simulink model "inverter_hil"  (R2024b)
settings: Solver=FixedStepDiscrete  StartTime=0.0  StopTime=inf  FixedStep=0.001  RelTol=1e-3
InitFcn:
  | enforceHardwarePreflight(bdroot);
values from neighbouring files (symbols this model uses):
  hil_cal_pedals_pressed_v1 = 1.1631952391851683    [inverter_hil.sldd]
  hil_cal_pedals_pressed_v2 = 2.341496910048066    [inverter_hil.sldd]
  hil_cal_pedals_pressed_v3 = 1.6012817578393226    [inverter_hil.sldd]
  hil_cal_pedals_pressed_v4 = 1.6012817578393226    [inverter_hil.sldd]
  hil_cal_pedals_released_v1 = 1.5156786449988555    [inverter_hil.sldd]
  hil_cal_pedals_released_v2 = 3.2025635156786452    [inverter_hil.sldd]
  hil_cal_pedals_released_v3 = 0.45445181963836118    [inverter_hil.sldd]
  hil_cal_pedals_released_v4 = 0.45445181963836118    [inverter_hil.sldd]
  hil_cmd_can_drop_control_mask = 0    [inverter_hil.sldd]
  hil_cmd_can_drop_status_mask = 0    [inverter_hil.sldd]
  hil_cmd_dc_link12_v = 0.0    [inverter_hil.sldd]
  hil_cmd_dc_link34_v = 0.0    [inverter_hil.sldd]
  hil_cmd_digital_cooling_switch = 0    [inverter_hil.sldd]
  hil_cmd_digital_main_button = 0    [inverter_hil.sldd]
  hil_cmd_digital_main_button_sequence = 0    [inverter_hil.sldd]
  hil_cmd_digital_precharge_sequence = 0    [inverter_hil.sldd]
  hil_cmd_digital_shutdown_feedback = 0    [inverter_hil.sldd]
  hil_cmd_gui_heartbeat = 0    [inverter_hil.sldd]
  hil_cmd_imu_dropout = 0    [inverter_hil.sldd]
  hil_cmd_imu_malformed = 0    [inverter_hil.sldd]
  hil_cmd_imu_stale = 0    [inverter_hil.sldd]
  hil_cmd_inverter1_connected = 1    [inverter_hil.sldd]
  hil_cmd_inverter1_fault_mask = 0    [inverter_hil.sldd]
  hil_cmd_inverter1_load_nm = 0.0    [inverter_hil.sldd]
  hil_cmd_inverter2_connected = 1    [inverter_hil.sldd]
  hil_cmd_inverter2_fault_mask = 0    [inverter_hil.sldd]
  hil_cmd_inverter2_load_nm = 0.0    [inverter_hil.sldd]
  hil_cmd_inverter3_connected = 1    [inverter_hil.sldd]
  hil_cmd_inverter3_fault_mask = 0    [inverter_hil.sldd]
  hil_cmd_inverter3_load_nm = 0.0    [inverter_hil.sldd]
  hil_cmd_inverter4_connected = 1    [inverter_hil.sldd]
  hil_cmd_inverter4_fault_mask = 0    [inverter_hil.sldd]
  hil_cmd_inverter4_load_nm = 0.0    [inverter_hil.sldd]
  hil_cmd_pedals_brake = 0.0    [inverter_hil.sldd]
  hil_cmd_pedals_plausibility_override = 0    [inverter_hil.sldd]
  hil_cmd_pedals_throttle = 0.0    [inverter_hil.sldd]
  hil_cmd_steering_angle_deg = 0.0    [inverter_hil.sldd]
  hil_cmd_steering_angle_sentinel = 0    [inverter_hil.sldd]
  hil_cmd_steering_calibration_sequence = 0    [inverter_hil.sldd]
  hil_cmd_steering_dropout = 0    [inverter_hil.sldd]
  hil_cmd_steering_invalid_status = 0    [inverter_hil.sldd]
  hil_cmd_steering_malformed = 0    [inverter_hil.sldd]
  hil_cmd_steering_speed_sentinel = 0    [inverter_hil.sldd]
  hil_cmd_steering_stale = 0    [inverter_hil.sldd]
undefined symbols (not defined in the file or in its folder): Pull, up
libraries: speedgoatlib_IO614 x21, canmsglib x16, speedgoatlib_IO183 x5
(part 1 of 3)
settings Model: DataDictionary=inverter_hil.sldd  Creator=MFE-HPC  LastModifiedBy=MFE-HPC
settings SolverCC: ConcurrentTasks=on  PositivePriorityOrder=on
settings OptimizationCC: BlockReduction=off  OptimizeBlockIOStorage=off
settings DebuggingCC: TasksWithSamePriorityMsg=none
settings HardwareCC: ProdBitPerLong=64  ProdLongLongMode=on  ProdHWDeviceType=Intel->x86-64 (Linux 64)
settings RTWCC: Description=Speedgoat Real-Time Target Machine  SystemTargetFile=speedgoat.tlc  TemplateMakefile=slrealtime_default_tmf  Toolchain=Simulink Real-Time Toolchain  BuildConfiguration=Faster Runs  CodeExecutionProfiling=on  TargetLang=C++
settings SimulinkRealTimeTargetCC: InstructionSetFMA=off  LogToMDFFile=off

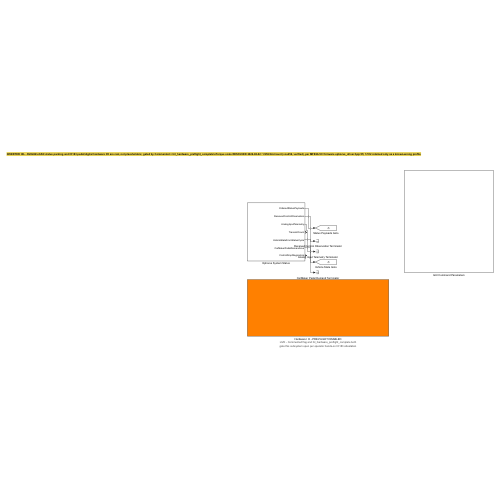
[thumbnail: Simulink's stored preview of the top-level diagram]
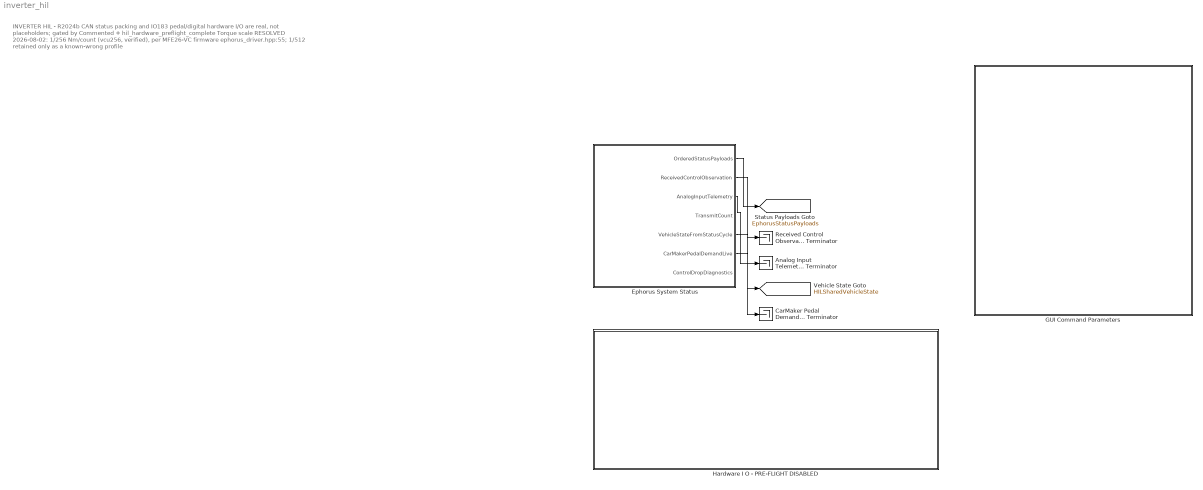
== system inverter_hil ==
  note: INVERTER HIL - R2024b\nCAN status packing and IO183 pedal/digital hardware I/O are real, not placeholders; gated by Commented + hil_hardware_preflight_complete\nTorque scale RESOLVED 2026-08-02: 1/256 Nm/count (vcu256, verified), per MFE26-VC firmware ephorus_driver.hpp:55; 1/512 retained only as a known-wrong profile
  Analog Input Telemetry Terminator : Terminator
  CarMaker Pedal Demand Terminator : Terminator
  Ephorus System Status : Subsystem
  GUI Command Parameters : Subsystem
  Hardware I O - PRE-FLIGHT DISABLED : Subsystem
      settings: AttributesFormatString=LIVE - Commented flag and hil_hardware_preflight_complete both\ngate this subsystem open per operator hands-on IO183 attestation
  Received Control Observation Terminator : Terminator
  tag scope: EphorusStatusPayloads=global, HILSharedVehicleState=global
  wires:
  Ephorus System Status/1(OrderedStatusPayloads) -> [EphorusStatusPayloads]
  Ephorus System Status/2(ReceivedControlObservation) -> Received Control Observation Terminator/1
  Ephorus System Status/3(AnalogInputTelemetry) -> Analog Input Telemetry Terminator/1
  Ephorus System Status/5(VehicleStateFromStatusCycle) -> [HILSharedVehicleState]
  Ephorus System Status/6(CarMakerPedalDemandLive) -> CarMaker Pedal Demand Terminator/1

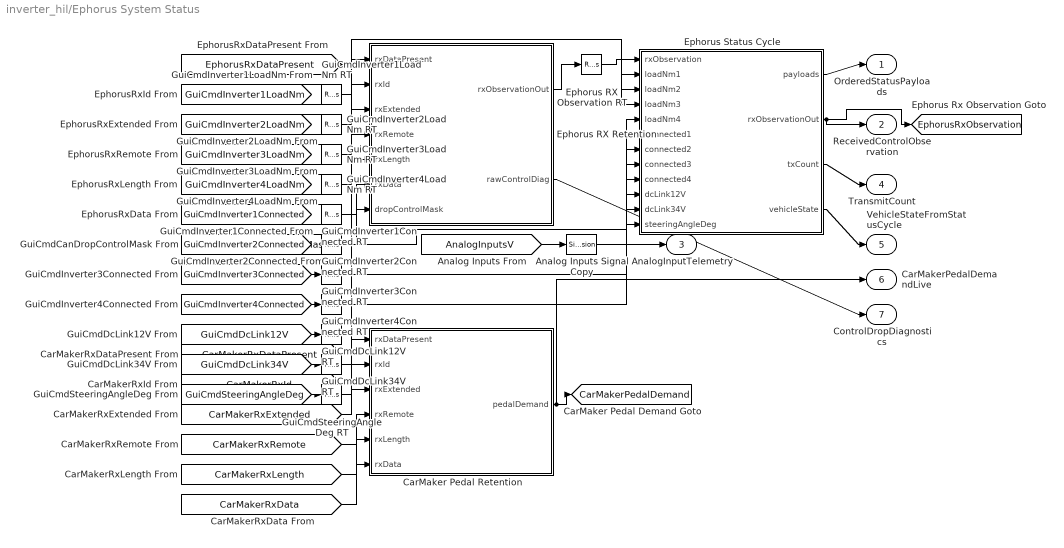
== system inverter_hil/Ephorus System Status ==
  Analog Inputs Signal Copy : SignalConversion  OverrideOpt=off
  CarMaker Pedal Retention : MATLAB Function  TreatAsAtomicUnit=on
  Ephorus RX Observation RT : RateTransition
  Ephorus RX Retention : MATLAB Function  TreatAsAtomicUnit=on
  Ephorus Status Cycle : MATLAB Function  TreatAsAtomicUnit=on
  GuiCmdDcLink12V RT : RateTransition
  GuiCmdDcLink34V RT : RateTransition
  GuiCmdInverter1Connected RT : RateTransition
  GuiCmdInverter1LoadNm RT : RateTransition
  GuiCmdInverter2Connected RT : RateTransition
  GuiCmdInverter2LoadNm RT : RateTransition
  GuiCmdInverter3Connected RT : RateTransition
  GuiCmdInverter3LoadNm RT : RateTransition
  GuiCmdInverter4Connected RT : RateTransition
  GuiCmdInverter4LoadNm RT : RateTransition
  GuiCmdSteeringAngleDeg RT : RateTransition
  OrderedStatusPayloads : Outport
  ReceivedControlObservation : Outport  Port=2
  AnalogInputTelemetry : Outport  Port=3
  TransmitCount : Outport  Port=4
  VehicleStateFromStatusCycle : Outport  Port=5
  CarMakerPedalDemandLive : Outport  Port=6
  ControlDropDiagnostics : Outport  Port=7
  tag scope: CarMakerPedalDemand=global, EphorusRxObservation=global
  wires:
  ? -> ?
  [EphorusRxDataPresent] -> Ephorus RX Retention/1(rxDataPresent)
  [EphorusRxId] -> Ephorus RX Retention/2(rxId)
  [EphorusRxExtended] -> Ephorus RX Retention/3(rxExtended)
  [EphorusRxRemote] -> Ephorus RX Retention/4(rxRemote)
  [EphorusRxLength] -> Ephorus RX Retention/5(rxLength)
  [EphorusRxData] -> Ephorus RX Retention/6(rxData)
  [GuiCmdCanDropControlMask] -> Ephorus RX Retention/7(dropControlMask)
  [CarMakerRxDataPresent] -> CarMaker Pedal Retention/1(rxDataPresent)
  [CarMakerRxId] -> CarMaker Pedal Retention/2(rxId)
  [CarMakerRxExtended] -> CarMaker Pedal Retention/3(rxExtended)
  [CarMakerRxRemote] -> CarMaker Pedal Retention/4(rxRemote)
  [CarMakerRxLength] -> CarMaker Pedal Retention/5(rxLength)
  [CarMakerRxData] -> CarMaker Pedal Retention/6(rxData)
  CarMaker Pedal Retention/1(pedalDemand) -> [CarMakerPedalDemand], CarMakerPedalDemandLive/1
  Ephorus RX Retention/1(rxObservationOut) -> Ephorus RX Observation RT/1
  Ephorus RX Observation RT/1 -> Ephorus Status Cycle/1(rxObservation)
  Ephorus Status Cycle/1(payloads) -> OrderedStatusPayloads/1
  Ephorus Status Cycle/2(rxObservationOut) -> ReceivedControlObservation/1, [EphorusRxObservation]
  Ephorus RX Retention/2(rawControlDiag) -> ControlDropDiagnostics/1
  [AnalogInputsV] -> Analog Inputs Signal Copy/1
  Analog Inputs Signal Copy/1 -> AnalogInputTelemetry/1
  Ephorus Status Cycle/3(txCount) -> TransmitCount/1
  Ephorus Status Cycle/4(vehicleState) -> VehicleStateFromStatusCycle/1
  [GuiCmdInverter1LoadNm] -> GuiCmdInverter1LoadNm RT/1
  GuiCmdInverter1LoadNm RT/1 -> Ephorus Status Cycle/2(loadNm1)
  [GuiCmdInverter2LoadNm] -> GuiCmdInverter2LoadNm RT/1
  GuiCmdInverter2LoadNm RT/1 -> Ephorus Status Cycle/3(loadNm2)
  [GuiCmdInverter3LoadNm] -> GuiCmdInverter3LoadNm RT/1
  GuiCmdInverter3LoadNm RT/1 -> Ephorus Status Cycle/4(loadNm3)
  [GuiCmdInverter4LoadNm] -> GuiCmdInverter4LoadNm RT/1
  GuiCmdInverter4LoadNm RT/1 -> Ephorus Status Cycle/5(loadNm4)
  [GuiCmdInverter1Connected] -> GuiCmdInverter1Connected RT/1
  GuiCmdInverter1Connected RT/1 -> Ephorus Status Cycle/6(connected1)
  [GuiCmdInverter2Connected] -> GuiCmdInverter2Connected RT/1
  GuiCmdInverter2Connected RT/1 -> Ephorus Status Cycle/7(connected2)
  [GuiCmdInverter3Connected] -> GuiCmdInverter3Connected RT/1
  GuiCmdInverter3Connected RT/1 -> Ephorus Status Cycle/8(connected3)
  [GuiCmdInverter4Connected] -> GuiCmdInverter4Connected RT/1
  GuiCmdInverter4Connected RT/1 -> Ephorus Status Cycle/9(connected4)
  [GuiCmdDcLink12V] -> GuiCmdDcLink12V RT/1
  GuiCmdDcLink12V RT/1 -> Ephorus Status Cycle/10(dcLink12V)
  [GuiCmdDcLink34V] -> GuiCmdDcLink34V RT/1
  GuiCmdDcLink34V RT/1 -> Ephorus Status Cycle/11(dcLink34V)
  [GuiCmdSteeringAngleDeg] -> GuiCmdSteeringAngleDeg RT/1
  GuiCmdSteeringAngleDeg RT/1 -> Ephorus Status Cycle/12(steeringAngleDeg)

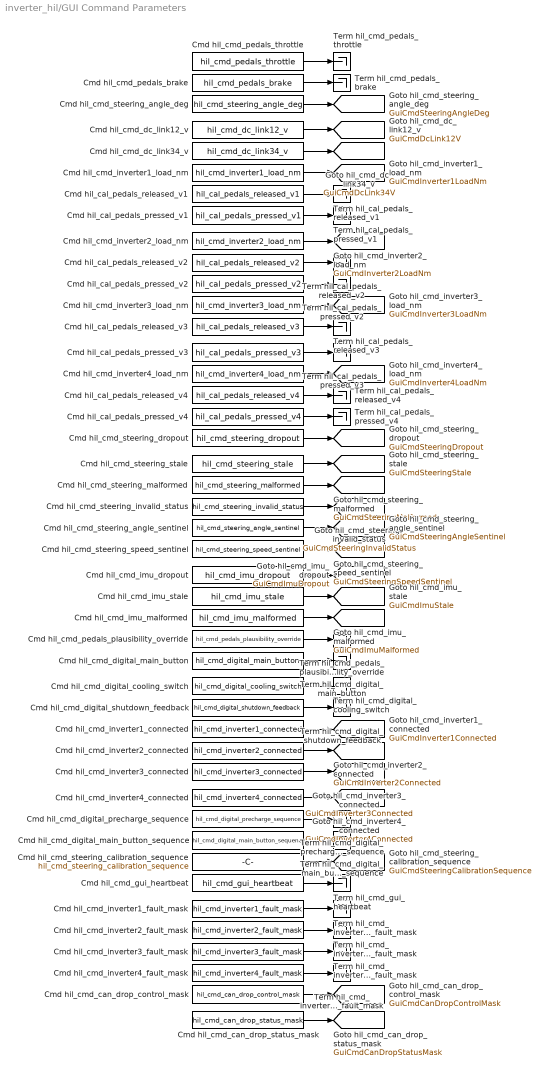
== system inverter_hil/GUI Command Parameters ==
  Cmd hil_cal_pedals_pressed_v1 : Constant  Value=hil_cal_pedals_pressed_v1  SampleTime=0.001
  Cmd hil_cal_pedals_pressed_v2 : Constant  Value=hil_cal_pedals_pressed_v2  SampleTime=0.001
  Cmd hil_cal_pedals_pressed_v3 : Constant  Value=hil_cal_pedals_pressed_v3  SampleTime=0.001
  Cmd hil_cal_pedals_pressed_v4 : Constant  Value=hil_cal_pedals_pressed_v4  SampleTime=0.001
  Cmd hil_cal_pedals_released_v1 : Constant  Value=hil_cal_pedals_released_v1  SampleTime=0.001
  Cmd hil_cal_pedals_released_v2 : Constant  Value=hil_cal_pedals_released_v2  SampleTime=0.001
  Cmd hil_cal_pedals_released_v3 : Constant  Value=hil_cal_pedals_released_v3  SampleTime=0.001
  Cmd hil_cal_pedals_released_v4 : Constant  Value=hil_cal_pedals_released_v4  SampleTime=0.001
  Cmd hil_cmd_can_drop_control_mask : Constant  Value=hil_cmd_can_drop_control_mask  OutDataTypeStr=uint8  SampleTime=0.001
  Cmd hil_cmd_can_drop_status_mask : Constant  Value=hil_cmd_can_drop_status_mask  OutDataTypeStr=uint16  SampleTime=0.001
  Cmd hil_cmd_dc_link12_v : Constant  Value=hil_cmd_dc_link12_v  SampleTime=0.001
  Cmd hil_cmd_dc_link34_v : Constant  Value=hil_cmd_dc_link34_v  SampleTime=0.001
  Cmd hil_cmd_digital_cooling_switch : Constant  Value=hil_cmd_digital_cooling_switch  OutDataTypeStr=boolean  SampleTime=0.001
  Cmd hil_cmd_digital_main_button : Constant  Value=hil_cmd_digital_main_button  OutDataTypeStr=boolean  SampleTime=0.001
  Cmd hil_cmd_digital_main_button_sequence : Constant  Value=hil_cmd_digital_main_button_sequence  OutDataTypeStr=uint32  SampleTime=0.001
  Cmd hil_cmd_digital_precharge_sequence : Constant  Value=hil_cmd_digital_precharge_sequence  OutDataTypeStr=uint32  SampleTime=0.001
  Cmd hil_cmd_digital_shutdown_feedback : Constant  Value=hil_cmd_digital_shutdown_feedback  OutDataTypeStr=boolean  SampleTime=0.001
  Cmd hil_cmd_gui_heartbeat : Constant  Value=hil_cmd_gui_heartbeat  OutDataTypeStr=uint32  SampleTime=0.001
  Cmd hil_cmd_imu_dropout : Constant  Value=hil_cmd_imu_dropout  OutDataTypeStr=boolean  SampleTime=0.001
  Cmd hil_cmd_imu_malformed : Constant  Value=hil_cmd_imu_malformed  OutDataTypeStr=boolean  SampleTime=0.001
  Cmd hil_cmd_imu_stale : Constant  Value=hil_cmd_imu_stale  OutDataTypeStr=boolean  SampleTime=0.001
  Cmd hil_cmd_inverter1_connected : Constant  Value=hil_cmd_inverter1_connected  OutDataTypeStr=boolean  SampleTime=0.001
  Cmd hil_cmd_inverter1_fault_mask : Constant  Value=hil_cmd_inverter1_fault_mask  OutDataTypeStr=uint32  SampleTime=0.001
  Cmd hil_cmd_inverter1_load_nm : Constant  Value=hil_cmd_inverter1_load_nm  SampleTime=0.001
  Cmd hil_cmd_inverter2_connected : Constant  Value=hil_cmd_inverter2_connected  OutDataTypeStr=boolean  SampleTime=0.001
  Cmd hil_cmd_inverter2_fault_mask : Constant  Value=hil_cmd_inverter2_fault_mask  OutDataTypeStr=uint32  SampleTime=0.001
  Cmd hil_cmd_inverter2_load_nm : Constant  Value=hil_cmd_inverter2_load_nm  SampleTime=0.001
  Cmd hil_cmd_inverter3_connected : Constant  Value=hil_cmd_inverter3_connected  OutDataTypeStr=boolean  SampleTime=0.001
  Cmd hil_cmd_inverter3_fault_mask : Constant  Value=hil_cmd_inverter3_fault_mask  OutDataTypeStr=uint32  SampleTime=0.001
  Cmd hil_cmd_inverter3_load_nm : Constant  Value=hil_cmd_inverter3_load_nm  SampleTime=0.001
  Cmd hil_cmd_inverter4_connected : Constant  Value=hil_cmd_inverter4_connected  OutDataTypeStr=boolean  SampleTime=0.001
  Cmd hil_cmd_inverter4_fault_mask : Constant  Value=hil_cmd_inverter4_fault_mask  OutDataTypeStr=uint32  SampleTime=0.001
  Cmd hil_cmd_inverter4_load_nm : Constant  Value=hil_cmd_inverter4_load_nm  SampleTime=0.001
  Cmd hil_cmd_pedals_brake : Constant  Value=hil_cmd_pedals_brake  SampleTime=0.001
  Cmd hil_cmd_pedals_plausibility_override : Constant  Value=hil_cmd_pedals_plausibility_override  OutDataTypeStr=boolean  SampleTime=0.001
  Cmd hil_cmd_pedals_throttle : Constant  Value=hil_cmd_pedals_throttle  SampleTime=0.001
  Cmd hil_cmd_steering_angle_deg : Constant  Value=hil_cmd_steering_angle_deg  SampleTime=0.001
  Cmd hil_cmd_steering_angle_sentinel : Constant  Value=hil_cmd_steering_angle_sentinel  OutDataTypeStr=boolean  SampleTime=0.001
  Cmd hil_cmd_steering_calibration_sequence : Constant  Value=hil_cmd_steering_calibration_sequence  OutDataTypeStr=uint32  SampleTime=0.001
  Cmd hil_cmd_steering_dropout : Constant  Value=hil_cmd_steering_dropout  OutDataTypeStr=boolean  SampleTime=0.001
  Cmd hil_cmd_steering_invalid_status : Constant  Value=hil_cmd_steering_invalid_status  OutDataTypeStr=boolean  SampleTime=0.001
  Cmd hil_cmd_steering_malformed : Constant  Value=hil_cmd_steering_malformed  OutDataTypeStr=boolean  SampleTime=0.001
  Cmd hil_cmd_steering_speed_sentinel : Constant  Value=hil_cmd_steering_speed_sentinel  OutDataTypeStr=boolean  SampleTime=0.001
  Cmd hil_cmd_steering_stale : Constant  Value=hil_cmd_steering_stale  OutDataTypeStr=boolean  SampleTime=0.001
  Term hil_cal_pedals_pressed_v{1..4} (4 alike) : Terminator
  Term hil_cal_pedals_released_v{1..4} (4 alike) : Terminator
  Term hil_cmd_digital_cooling_switch : Terminator
  Term hil_cmd_digital_main_button : Terminator
  Term hil_cmd_digital_main_button_sequence : Terminator
  Term hil_cmd_digital_precharge_sequence : Terminator
  Term hil_cmd_digital_shutdown_feedback : Terminator
  Term hil_cmd_gui_heartbeat : Terminator
  Term hil_cmd_inverter1_fault_mask : Terminator
  Term hil_cmd_inverter2_fault_mask : Terminator
  Term hil_cmd_inverter3_fault_mask : Terminator
  Term hil_cmd_inverter4_fault_mask : Terminator
  Term hil_cmd_pedals_brake : Terminator
  Term hil_cmd_pedals_plausibility_override : Terminator
  Term hil_cmd_pedals_throttle : Terminator
  tag scope: GuiCmdCanDropControlMask=global, GuiCmdCanDropStatusMask=global, GuiCmdDcLink12V=global, GuiCmdDcLink34V=global, GuiCmdImuDropout=global, GuiCmdImuMalformed=global, GuiCmdImuStale=global, GuiCmdInverter1Connected=global, GuiCmdInverter1LoadNm=global, GuiCmdInverter2Connected=global, GuiCmdInverter2LoadNm=global, GuiCmdInverter3Connected=global, GuiCmdInverter3LoadNm=global, GuiCmdInverter4Connected=global, GuiCmdInverter4LoadNm=global, GuiCmdSteeringAngleDeg=global, GuiCmdSteeringAngleSentinel=global, GuiCmdSteeringCalibrationSequence=global, GuiCmdSteeringDropout=global, GuiCmdSteeringInvalidStatus=global, GuiCmdSteeringMalformed=global, GuiCmdSteeringSpeedSentinel=global, GuiCmdSteeringStale=global
  wires:
  ? -> ?
  Cmd hil_cmd_pedals_throttle/1 -> Term hil_cmd_pedals_throttle/1
  Cmd hil_cmd_pedals_brake/1 -> Term hil_cmd_pedals_brake/1
  Cmd hil_cmd_steering_angle_deg/1 -> [GuiCmdSteeringAngleDeg]
  Cmd hil_cmd_dc_link12_v/1 -> [GuiCmdDcLink12V]
  Cmd hil_cmd_dc_link34_v/1 -> [GuiCmdDcLink34V]
  Cmd hil_cmd_inverter1_load_nm/1 -> [GuiCmdInverter1LoadNm]
  Cmd hil_cal_pedals_released_v1/1 -> Term hil_cal_pedals_released_v1/1
  Cmd hil_cal_pedals_pressed_v1/1 -> Term hil_cal_pedals_pressed_v1/1
  Cmd hil_cmd_inverter2_load_nm/1 -> [GuiCmdInverter2LoadNm]
  Cmd hil_cal_pedals_released_v2/1 -> Term hil_cal_pedals_released_v2/1
  Cmd hil_cal_pedals_pressed_v2/1 -> Term hil_cal_pedals_pressed_v2/1
  Cmd hil_cmd_inverter3_load_nm/1 -> [GuiCmdInverter3LoadNm]
  Cmd hil_cal_pedals_released_v3/1 -> Term hil_cal_pedals_released_v3/1
  Cmd hil_cal_pedals_pressed_v3/1 -> Term hil_cal_pedals_pressed_v3/1
  Cmd hil_cmd_inverter4_load_nm/1 -> [GuiCmdInverter4LoadNm]
  Cmd hil_cal_pedals_released_v4/1 -> Term hil_cal_pedals_released_v4/1
  Cmd hil_cal_pedals_pressed_v4/1 -> Term hil_cal_pedals_pressed_v4/1
  Cmd hil_cmd_steering_dropout/1 -> [GuiCmdSteeringDropout]
  Cmd hil_cmd_steering_stale/1 -> [GuiCmdSteeringStale]
  Cmd hil_cmd_steering_malformed/1 -> [GuiCmdSteeringMalformed]
  Cmd hil_cmd_steering_invalid_status/1 -> [GuiCmdSteeringInvalidStatus]
  Cmd hil_cmd_steering_angle_sentinel/1 -> [GuiCmdSteeringAngleSentinel]
  Cmd hil_cmd_steering_speed_sentinel/1 -> [GuiCmdSteeringSpeedSentinel]
  Cmd hil_cmd_imu_dropout/1 -> [GuiCmdImuDropout]
  Cmd hil_cmd_imu_stale/1 -> [GuiCmdImuStale]
  Cmd hil_cmd_imu_malformed/1 -> [GuiCmdImuMalformed]
  Cmd hil_cmd_pedals_plausibility_override/1 -> Term hil_cmd_pedals_plausibility_override/1
  Cmd hil_cmd_digital_main_button/1 -> Term hil_cmd_digital_main_button/1
  Cmd hil_cmd_digital_cooling_switch/1 -> Term hil_cmd_digital_cooling_switch/1
  Cmd hil_cmd_digital_shutdown_feedback/1 -> Term hil_cmd_digital_shutdown_feedback/1
  Cmd hil_cmd_inverter1_connected/1 -> [GuiCmdInverter1Connected]
  Cmd hil_cmd_inverter2_connected/1 -> [GuiCmdInverter2Connected]
  Cmd hil_cmd_inverter3_connected/1 -> [GuiCmdInverter3Connected]
  Cmd hil_cmd_inverter4_connected/1 -> [GuiCmdInverter4Connected]
  Cmd hil_cmd_digital_precharge_sequence/1 -> Term hil_cmd_digital_precharge_sequence/1
  Cmd hil_cmd_digital_main_button_sequence/1 -> Term hil_cmd_digital_main_button_sequence/1
  Cmd hil_cmd_steering_calibration_sequence/1 -> [GuiCmdSteeringCalibrationSequence]
  Cmd hil_cmd_gui_heartbeat/1 -> Term hil_cmd_gui_heartbeat/1
  Cmd hil_cmd_inverter1_fault_mask/1 -> Term hil_cmd_inverter1_fault_mask/1
  Cmd hil_cmd_inverter2_fault_mask/1 -> Term hil_cmd_inverter2_fault_mask/1
  Cmd hil_cmd_inverter3_fault_mask/1 -> Term hil_cmd_inverter3_fault_mask/1
  Cmd hil_cmd_inverter4_fault_mask/1 -> Term hil_cmd_inverter4_fault_mask/1
  Cmd hil_cmd_can_drop_control_mask/1 -> [GuiCmdCanDropControlMask]
  Cmd hil_cmd_can_drop_status_mask/1 -> [GuiCmdCanDropStatusMask]
